simulink model "ClosedLoopTest_v2"  (R2023a)
settings: Solver=VariableStepAuto  StartTime=0.0  StopTime=500  RelTol=1e-3
undefined symbols (not defined in the file): B, I, J, Ke, Kt, La, Ra, T_ext, T_max, T_max_mgt
libraries: matrix_library x4, simulink_extras x3, slpidlib x2, vrlib x2, aerolibutil x1
settings Model: Creator=Personal  LastModifiedBy=Personal

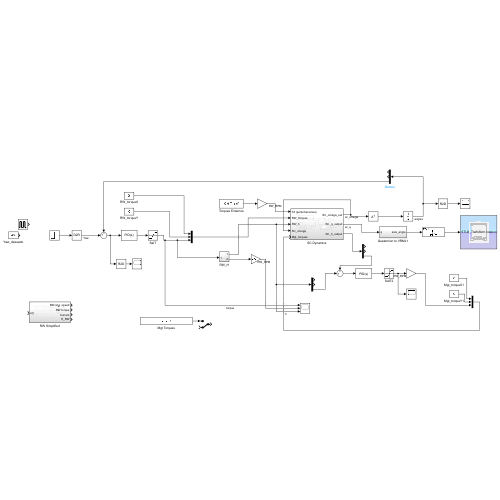
[thumbnail: Simulink's stored preview of the top-level diagram]
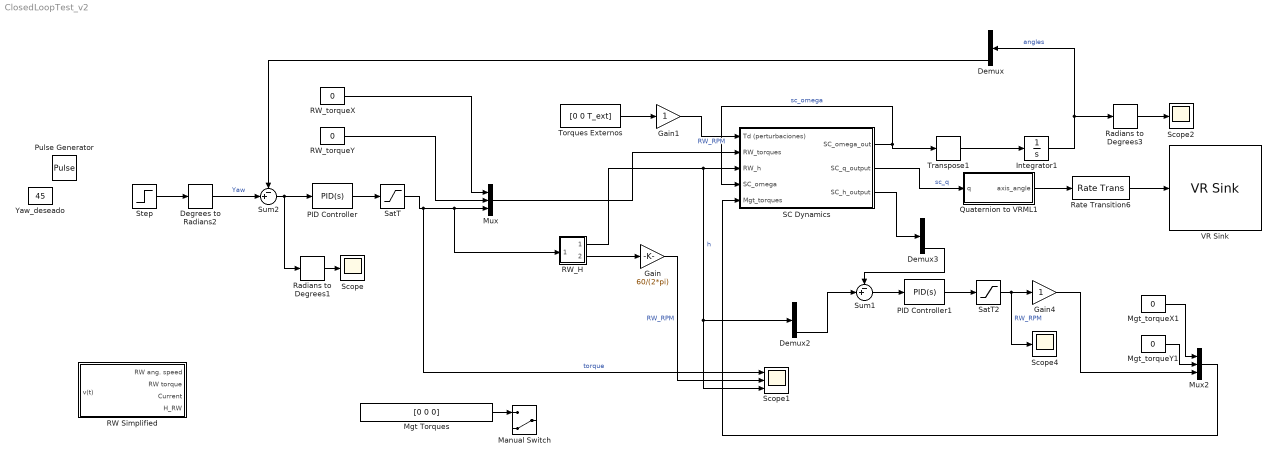
== system ClosedLoopTest_v2 ==
  Degrees to Radians2 : simulink_extras/Transformations/Degrees to Radians
  Demux : Demux  Outputs=3
  Demux2 : Demux  Outputs=3
  Demux3 : Demux  Outputs=3
  Gain : Gain  Gain=60/(2*pi)
  Gain1 : Gain
  Gain4 : Gain
  Integrator1 : Integrator  InitialCondition=[0 0 0]
  Manual Switch : ManualSwitch  CurrentSetting=0
  Mgt Torques : Constant  Value=[0 0 0]
  Mgt_torqueX1 : Constant  Value=0
  Mgt_torqueY1 : Constant  Value=0
  Mux : Mux  Inputs=3
  Mux2 : Mux  Inputs=3
  PID Controller : slpidlib/PID Controller  Controller=PID  Form=Parallel  TimeDomain=Continuous-time  UseExternalTs=off  SampleTime=-1  IntegratorMethod=Forward Euler  FilterMethod=Forward Euler  ControllerParametersSource=internal  P=4500  I=800  UseKiTs=off  D=8000  N=100  UseFilter=on  TunerSelectOption=Transfer Function Based (PID Tuner App)  InitialConditionSource=internal  InitialConditionForIntegrator=0  InitialConditionForFilter=0  DifferentiatorICPrevScaledInput=0  ExternalReset=none  TrackingMode=off  Kt=1  LimitOutput=off  SatLimitsSource=internal  UpperSaturationLimit=1  LowerSaturationLimit=-1  LinearizeAsGain=on  AntiWindupMode=none  Kb=1  LimitIntegrator=off  UpperIntegratorSaturationLimit=inf  LowerIntegratorSaturationLimit=-inf  POutMin=[]  POutMax=[]  IOutMin=[]  IOutMax=[]  DOutMin=[]  DOutMax=[]  NOutMin=[]  NOutMax=[]  SumOutMin=[]  SumOutMax=[]  SaturationOutMin=[]  SaturationOutMax=[]  PParamMin=[]  PParamMax=[]  IParamMin=[]  IParamMax=[]  DParamMin=[]  DParamMax=[]  NParamMin=[]  NParamMax=[]  KbParamMin=[]  KbParamMax=[]  KtParamMin=[]  KtParamMax=[]  KbOutMin=[]  KbOutMax=[]  KtOutMin=[]  KtOutMax=[]  IntegratorOutMin=[]  IntegratorOutMax=[]  FilterOutMin=[]  FilterOutMax=[]  SumI1OutMin=[]  SumI1OutMax=[]  SumI2OutMin=[]  SumI2OutMax=[]  SumI3OutMin=[]  SumI3OutMax=[]  SumI4OutMin=[]  SumI4OutMax=[]  SumDOutMin=[]  SumDOutMax=[]  DifferentiatorOutMin=[]  DifferentiatorOutMax=[]  FilterDiffOutCoefMin=[]  FilterDiffOutCoefMax=[]  ReciprocalOutMin=[]  ReciprocalOutMax=[]  SumDenOutMin=[]  SumDenOutMax=[]  SumNumOutMin=[]  SumNumOutMax=[]  DivideOutMin=[]  DivideOutMax=[]  UdiffTsProdOutMin=[]  UdiffTsProdOutMax=[]  NTsProdOutMin=[]  NTsProdOutMax=[]  UintegralTsProdOutMin=[]  UintegralTsProdOutMax=[]  UngainTsProdOutMin=[]  UngainTsProdOutMax=[]  ClampingZeroOutDataTypeStr=Inherit: Inherit via back propagation  ClampingZeroOutMin=[]  ClampingZeroOutMax=[]  FilterDenConstantOutDataTypeStr=Inherit: Inherit via back propagation  FilterDenConstantOutMin=[]  FilterDenConstantOutMax=[]  PCopyOutDataTypeStr=Inherit: Inherit via back propagation  PCopyOutMin=[]  PCopyOutMax=[]  NCopyOutDataTypeStr=Inherit: Inherit via back propagation  NCopyOutMin=[]  NCopyOutMax=[]  IntegratorContinuousStateAttributes=''  IntegratorStateMustResolveToSignalObject=off  IntegratorRTWStateStorageClass=Auto  FilterContinuousStateAttributes=''  FilterStateMustResolveToSignalObject=off  FilterRTWStateStorageClass=Auto  ParallelPVariant=InternalParameters  IdealPVariant=Disabled  IVariant=InternalParameters  DVariant=InternalParameters  IntegratorVariant=Continuous  SatVariant=Disabled  AWVariant=Passthrough  PCopyVariant=Disabled  TRVariant=Disabled  FdbkBlocksVariant=Forward  IdealPFdbkVariant=Disabled  SatFdbkVariant=Disabled  DerivativeFilterVariant=ContFilter  NVariant=InternalParameters  NCopyVariant=Disabled  FilterICVariant=InternalICsFilter  IntegratorICVariant=InternalICs  ExternalResetVariant=Disabled  TRSumVariant=Passthrough  SumFdbkVariant=Disabled  SumVariant=Sum_PID  TsampFilterVariant=InternalTs  TsampNgainVariant=Passthrough  TsampIntegralVariant=Disabled_SignalSpec  ExternalSaturationOutDataTypeStr=Inherit: Same as second input
  PID Controller1 : slpidlib/PID Controller  Controller=PID  Form=Parallel  TimeDomain=Continuous-time  UseExternalTs=off  SampleTime=-1  IntegratorMethod=Forward Euler  FilterMethod=Forward Euler  ControllerParametersSource=internal  P=4500  I=800  UseKiTs=off  D=8000  N=100  UseFilter=on  TunerSelectOption=Transfer Function Based (PID Tuner App)  InitialConditionSource=internal  InitialConditionForIntegrator=0  InitialConditionForFilter=0  DifferentiatorICPrevScaledInput=0  ExternalReset=none  TrackingMode=off  Kt=1  LimitOutput=off  SatLimitsSource=internal  UpperSaturationLimit=1  LowerSaturationLimit=-1  LinearizeAsGain=on  AntiWindupMode=none  Kb=1  LimitIntegrator=off  UpperIntegratorSaturationLimit=inf  LowerIntegratorSaturationLimit=-inf  POutMin=[]  POutMax=[]  IOutMin=[]  IOutMax=[]  DOutMin=[]  DOutMax=[]  NOutMin=[]  NOutMax=[]  SumOutMin=[]  SumOutMax=[]  SaturationOutMin=[]  SaturationOutMax=[]  PParamMin=[]  PParamMax=[]  IParamMin=[]  IParamMax=[]  DParamMin=[]  DParamMax=[]  NParamMin=[]  NParamMax=[]  KbParamMin=[]  KbParamMax=[]  KtParamMin=[]  KtParamMax=[]  KbOutMin=[]  KbOutMax=[]  KtOutMin=[]  KtOutMax=[]  IntegratorOutMin=[]  IntegratorOutMax=[]  FilterOutMin=[]  FilterOutMax=[]  SumI1OutMin=[]  SumI1OutMax=[]  SumI2OutMin=[]  SumI2OutMax=[]  SumI3OutMin=[]  SumI3OutMax=[]  SumI4OutMin=[]  SumI4OutMax=[]  SumDOutMin=[]  SumDOutMax=[]  DifferentiatorOutMin=[]  DifferentiatorOutMax=[]  FilterDiffOutCoefMin=[]  FilterDiffOutCoefMax=[]  ReciprocalOutMin=[]  ReciprocalOutMax=[]  SumDenOutMin=[]  SumDenOutMax=[]  SumNumOutMin=[]  SumNumOutMax=[]  DivideOutMin=[]  DivideOutMax=[]  UdiffTsProdOutMin=[]  UdiffTsProdOutMax=[]  NTsProdOutMin=[]  NTsProdOutMax=[]  UintegralTsProdOutMin=[]  UintegralTsProdOutMax=[]  UngainTsProdOutMin=[]  UngainTsProdOutMax=[]  ClampingZeroOutDataTypeStr=Inherit: Inherit via back propagation  ClampingZeroOutMin=[]  ClampingZeroOutMax=[]  FilterDenConstantOutDataTypeStr=Inherit: Inherit via back propagation  FilterDenConstantOutMin=[]  FilterDenConstantOutMax=[]  PCopyOutDataTypeStr=Inherit: Inherit via back propagation  PCopyOutMin=[]  PCopyOutMax=[]  NCopyOutDataTypeStr=Inherit: Inherit via back propagation  NCopyOutMin=[]  NCopyOutMax=[]  IntegratorContinuousStateAttributes=''  IntegratorStateMustResolveToSignalObject=off  IntegratorRTWStateStorageClass=Auto  FilterContinuousStateAttributes=''  FilterStateMustResolveToSignalObject=off  FilterRTWStateStorageClass=Auto  ParallelPVariant=InternalParameters  IdealPVariant=Disabled  IVariant=InternalParameters  DVariant=InternalParameters  IntegratorVariant=Continuous  SatVariant=Disabled  AWVariant=Passthrough  PCopyVariant=Disabled  TRVariant=Disabled  FdbkBlocksVariant=Forward  IdealPFdbkVariant=Disabled  SatFdbkVariant=Disabled  DerivativeFilterVariant=ContFilter  NVariant=InternalParameters  NCopyVariant=Disabled  FilterICVariant=InternalICsFilter  IntegratorICVariant=InternalICs  ExternalResetVariant=Disabled  TRSumVariant=Passthrough  SumFdbkVariant=Disabled  SumVariant=Sum_PID  TsampFilterVariant=InternalTs  TsampNgainVariant=Passthrough  TsampIntegralVariant=Disabled_SignalSpec  ExternalSaturationOutDataTypeStr=Inherit: Same as second input
  Pulse Generator : DiscretePulseGenerator  PulseType=Time based  Amplitude=45  Period=20  PulseWidth=50
  Quaternion to VRML1 : Subsystem
  RW Simplified : Subsystem
  RW_H : Subsystem
  RW_torqueX : Constant  Value=0
  RW_torqueY : Constant  Value=0
  Radians to Degrees1 : simulink_extras/Transformations/Radians to Degrees
  Radians to Degrees3 : simulink_extras/Transformations/Radians to Degrees
  Rate Transition6 : RateTransition
  SC Dynamics : Subsystem
  SatT : Saturate  UpperLimit=T_max  LowerLimit=-T_max
  SatT2 : Saturate  UpperLimit=T_max_mgt  LowerLimit=-T_max_mgt
  Scope : Scope
  Scope1 : Scope  NumInputPorts=3
  Scope2 : Scope
  Scope4 : Scope
  Step : Step  Time=5  After=90  SampleTime=0
  Sum1 : Sum  Inputs=-+|
  Sum2 : Sum  Inputs=-+|
  Torques Externos : Constant  Value=[0 0 T_ext]
  Transpose1 : matrix_library/Transpose
  VR Sink : vrlib/VR Sink  InstantiateOnLoad=on  SampleTime=0.1  ViewEnable=on  RemoteChange=off  RemoteView=off  FieldsWritten=STLB_Transform.rotation.4.1.1.double  WorldFileName=EscenarioCubeSat.x3d  AutoView=off  VideoDimensions=[]  AllowVariableSize=off
  Yaw_deseado : Constant  Value=45
  wires:
  Torques Externos/1 -> Gain1/1
  SC Dynamics/1(SC_omega_out) -> Transpose1/1, SC Dynamics/4(SC_omega)  "sc_omega"
  Degrees to Radians2/1 -> Sum2/2  "Yaw"
  Sum2/1 -> PID Controller/1, Radians to Degrees1/1
  Integrator1/1 -> Radians to Degrees3/1, Demux/1  "angles"
  Demux/3 -> Sum2/1
  PID Controller/1 -> SatT/1
  RW_torqueY/1 -> Mux/2
  RW_torqueX/1 -> Mux/1
  Mux/1 -> SC Dynamics/2(RW_torques)
  Step/1 -> Degrees to Radians2/1
  Transpose1/1 -> Integrator1/1
  SatT/1 -> Scope1/1, RW_H/1(In1), Mux/3  "torque"
  SC Dynamics/2(SC_q_output) -> Quaternion to VRML1/1(q)  "sc_q"
  Quaternion to VRML1/1(axis_angle) -> Rate Transition6/1
  Rate Transition6/1 -> VR Sink/1
  RW_H/1(Out1) -> Demux2/1, Scope1/3, SC Dynamics/3(RW_h)  "h"
  Radians to Degrees1/1 -> Scope/1
  Radians to Degrees3/1 -> Scope2/1
  RW_H/2(Out2) -> Gain/1
  Gain/1 -> Scope1/2  "RW_RPM"
  Gain1/1 -> SC Dynamics/1(Td (perturbaciones))  "RW_RPM"
  Mgt Torques/1 -> Manual Switch/1
  SC Dynamics/3(SC_h_output) -> Demux3/1
  Sum1/1 -> PID Controller1/1
  PID Controller1/1 -> SatT2/1
  Demux2/3 -> Sum1/2
  Demux3/3 -> Sum1/1
  Mgt_torqueX1/1 -> Mux2/1
  Mgt_torqueY1/1 -> Mux2/2
  SatT2/1 -> Scope4/1, Gain4/1  "RW_RPM"
  Mux2/1 -> SC Dynamics/5(Mgt_torques)
  Gain4/1 -> Mux2/3

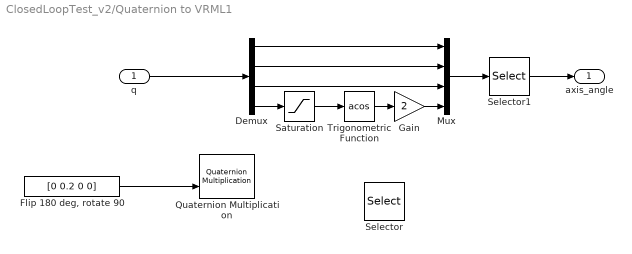
== system ClosedLoopTest_v2/Quaternion to VRML1 ==
  q : Inport
  Demux : Demux
  "Flip 180 deg, rotate 90" : Constant  Value=[0 0.2 0 0]
  Gain : Gain  Gain=2
  Mux : Mux
  Quaternion Multiplication : aerolibutil/Quaternion Multiplication
  Saturation : Saturate  UpperLimit=1  LowerLimit=-1  ZeroCross=off
  Selector : Selector  InputPortWidth=3  IndexOptions=Index vector (dialog)  Indices=[1 3]  OutputSizes=1
  Selector1 : Selector  InputPortWidth=4  IndexOptions=Index vector (dialog)  Indices=[2 3 1 4]  OutputSizes=1
  Trigonometric Function : Trigonometry  Operator=acos
  axis_angle : Outport  VectorParamsAs1DForOutWhenUnconnected=off
  wires:
  Demux/2 -> Mux/2
  "Flip 180 deg, rotate 90"/1 -> Quaternion Multiplication/2
  q/1 -> Demux/1
  Demux/1 -> Mux/1
  Mux/1 -> Selector1/1
  Selector1/1 -> axis_angle/1
  Trigonometric Function/1 -> Gain/1
  Gain/1 -> Mux/4
  Demux/3 -> Mux/3
  Saturation/1 -> Trigonometric Function/1
  Demux/4 -> Saturation/1

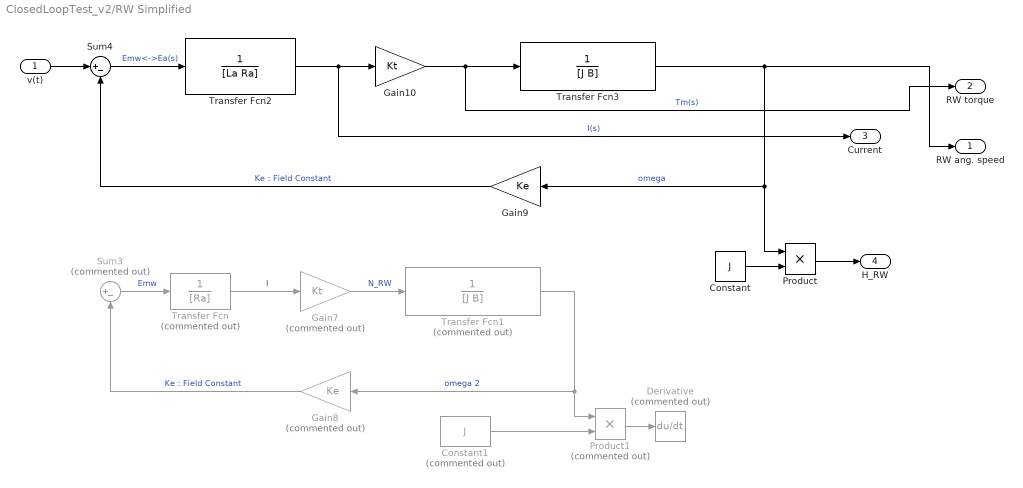
== system ClosedLoopTest_v2/RW Simplified ==
  v(t) : Inport
  Constant : Constant  Value=J
  Constant1 : Constant  Commented=on  Value=J
  Derivative : Derivative  Commented=on
  Gain10 : Gain  Gain=Kt
  Gain7 : Gain  Commented=on  Gain=Kt
  Gain8 : Gain  Commented=on  Gain=Ke
  Gain9 : Gain  Gain=Ke
  Product : Product
  Product1 : Product  Commented=on
  Sum3 : Sum  Commented=on  Inputs=|+-
  Sum4 : Sum  Inputs=|+-
  Transfer Fcn : TransferFcn  Commented=on  Denominator=[Ra]
  Transfer Fcn1 : TransferFcn  Commented=on  Denominator=[J B]
  Transfer Fcn2 : TransferFcn  Denominator=[La Ra]
  Transfer Fcn3 : TransferFcn  Denominator=[J B]
  RW ang. speed : Outport  VectorParamsAs1DForOutWhenUnconnected=off
  RW torque : Outport  Port=2  VectorParamsAs1DForOutWhenUnconnected=off
  Current : Outport  Port=3  VectorParamsAs1DForOutWhenUnconnected=off
  H_RW : Outport  Port=4  VectorParamsAs1DForOutWhenUnconnected=off
  wires:
  Gain10/1 -> RW torque/1, Transfer Fcn3/1  "Tm(s)"
  Transfer Fcn2/1 -> Current/1, Gain10/1  "I(s)"
  Sum4/1 -> Transfer Fcn2/1  "Emw<->Ea(s)"
  Gain9/1 -> Sum4/2  "Ke : Field Constant"
  Transfer Fcn3/1 -> Gain9/1, Product/1, RW ang. speed/1  "omega"
  Constant/1 -> Product/2
  Product/1 -> H_RW/1
  v(t)/1 -> Sum4/1
  Product1/1 -> Derivative/1
  Constant1/1 -> Product1/2
  Transfer Fcn1/1 -> Product1/1, Gain8/1  "omega 2"
  Gain7/1 -> Transfer Fcn1/1  "N_RW"
  Sum3/1 -> Transfer Fcn/1  "Emw"
  Transfer Fcn/1 -> Gain7/1  "I"
  Gain8/1 -> Sum3/2  "Ke : Field Constant"

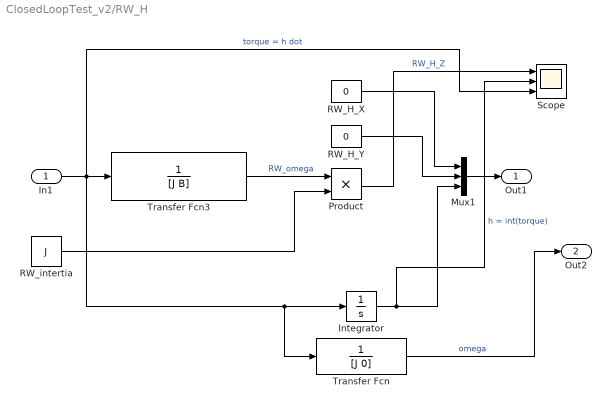
== system ClosedLoopTest_v2/RW_H ==
  In1 : Inport
  Integrator : Integrator
  Mux1 : Mux  Inputs=3
  Product : Product
  RW_H_X : Constant  Value=0
  RW_H_Y : Constant  Value=0
  RW_intertia : Constant  Value=J
  Scope : Scope  NumInputPorts=3
  Transfer Fcn : TransferFcn  Denominator=[J 0]
  Transfer Fcn3 : TransferFcn  Denominator=[J B]
  Out1 : Outport
  Out2 : Outport  Port=2
  wires:
  RW_H_Y/1 -> Mux1/2
  RW_intertia/1 -> Product/2
  In1/1 -> Scope/3, Transfer Fcn3/1, Transfer Fcn/1, Integrator/1  "torque = h dot"
  RW_H_X/1 -> Mux1/1
  Mux1/1 -> Out1/1
  Transfer Fcn3/1 -> Product/1  "RW_omega"
  Integrator/1 -> Scope/2, Mux1/3  "h = int(torque)"
  Transfer Fcn/1 -> Out2/1  "omega"
  Product/1 -> Scope/1  "RW_H_Z"

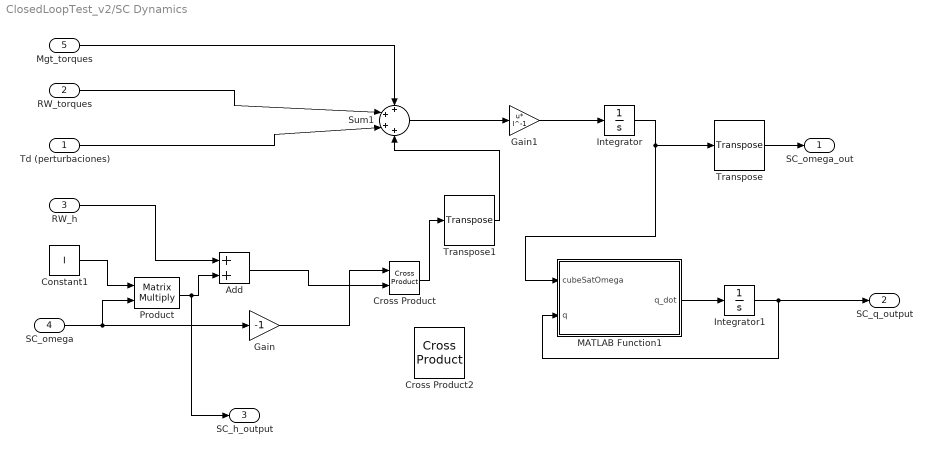
== system ClosedLoopTest_v2/SC Dynamics ==
  Td (perturbaciones) : Inport
  RW_torques : Inport  Port=2
  RW_h : Inport  Port=3
  SC_omega : Inport  Port=4
  Mgt_torques : Inport  Port=5
  Add : Sum
  Constant1 : Constant  Value=I
  Cross Product : vrlib/Utilities/Cross Product
  Cross Product2 : matrix_library/Cross Product
  Gain : Gain  Gain=-1
  Gain1 : Gain  Gain=I^-1  Multiplication=Matrix(u*K)
  Integrator : Integrator  InitialCondition=[0 0 0]
  Integrator1 : Integrator  InitialCondition=[0 0 0 1]
  MATLAB Function1 : MATLAB Function  TreatAsAtomicUnit=on
  Product : Product  Multiplication=Matrix(*)
  Sum1 : Sum  Inputs=++++
  Transpose : matrix_library/Transpose
  Transpose1 : matrix_library/Transpose
  SC_omega_out : Outport
  SC_q_output : Outport  Port=2
  SC_h_output : Outport  Port=3
  wires:
  RW_torques/1 -> Sum1/2
  Td (perturbaciones)/1 -> Sum1/3
  Integrator1/1 -> MATLAB Function1/2(q), SC_q_output/1
  Constant1/1 -> Product/1
  Product/1 -> SC_h_output/1, Add/2
  RW_h/1 -> Add/1
  Gain/1 -> Cross Product/1
  Add/1 -> Cross Product/2
  Cross Product/1 -> Transpose1/1
  Sum1/1 -> Gain1/1
  Gain1/1 -> Integrator/1
  Integrator/1 -> MATLAB Function1/1(cubeSatOmega), Transpose/1
  MATLAB Function1/1(q_dot) -> Integrator1/1
  Mgt_torques/1 -> Sum1/1
  SC_omega/1 -> Product/2, Gain/1
  Transpose/1 -> SC_omega_out/1
  Transpose1/1 -> Sum1/4

== matlab function ClosedLoopTest_v2/SC Dynamics/MATLAB Function1 ==
  data: cubeSatOmega input; q_dot output; q input
function q_dot = omega2qdot(cubeSatOmega,q)

wx = cubeSatOmega(1);
wy = cubeSatOmega(2);
wz = cubeSatOmega(3);

OmegaMatrix = [0 wz -wy wx ;
               -wz 0 wx wy; 
               wy -wx 0 wz;
               -wx -wy -wz 0];
            
q_dot=0.5*OmegaMatrix*q;

end
